simulink model "model_Asy_Motor_Control_PWM_v1"  (R2017b)
settings: Solver=ode45  StartTime=0.0  StopTime=3  MaxStep=1e-4  RelTol=1e-3
libraries: powerlib x8, dspstat3 x2, powerlib_meascontrol x1, simulink x1
settings Model: SimulationMode=accelerator  Creator=proso  LastModifiedBy=proso

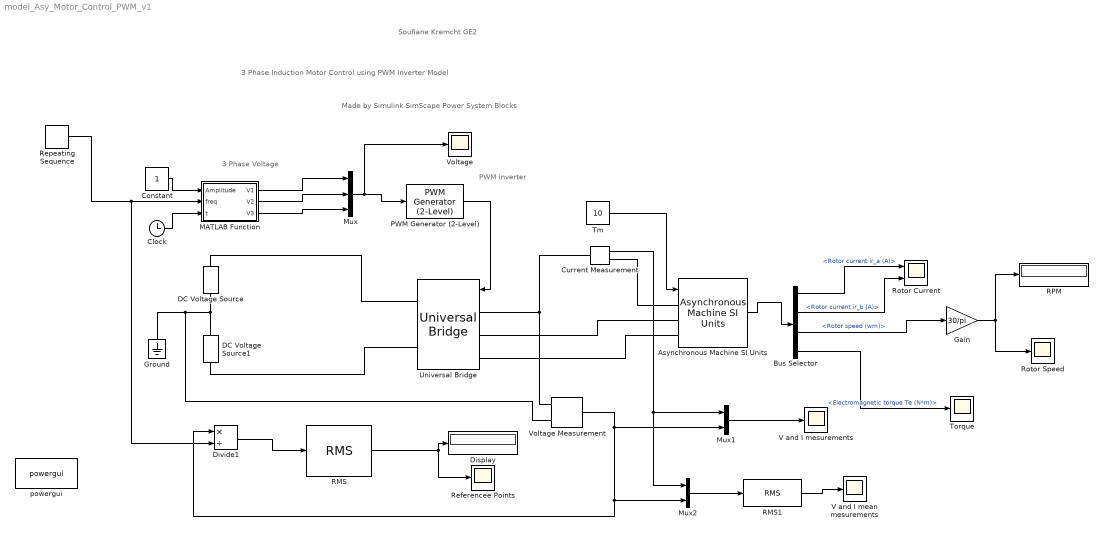
== system model_Asy_Motor_Control_PWM_v1 ==
  note: 3 Phase Voltage
  note: PWM inverter
  note: Soufiane Kremcht GE2
  note: Made by Simulink SimScape Power System Blocks
  note: 3 Phase Induction Motor Control using PWM Inverter Model
  Asynchronous Machine SI Units : powerlib/Machines/Asynchronous Machine SI Units  RotorType=Squirrel-cage  PresetModel="15:  5.4 HP (4KW)   400 V  50Hz 1430 RPM"  MechanicalLoad=Torque Tm  ShowDetailedParameters=on  ReferenceFrame=Rotor  Units=SI  MeasurementBus=off  NominalParameters=[4000 400 50]  Stator=[1.405 0.005839]  Rotor=[1.395 0.005839]  Cage1=[1.543 0.006067]  Cage2=[3.309 0.005654]  Lm=0.1722  Mechanical=[0.0131 0.002985 2]  PolePairs=2  InitialConditions=[0 0 0 0 0 0 0 0]  SimulateSaturation=off  Saturation=[14.03593122, 27.81365428, 53.79336849, 72.68890987, 97.98006896, 148.6815601, 215.7428561, 302.9841135, 428.7778367 ; 230, 322, 414, 460, 506, 552, 598, 644, 690]  LoadFlowParameters=1492000  TsPowergui=0  TsBlock=-1  IterativeModel=Trapezoidal non iterative  IterativeDiscreteModel=Trapezoidal non iterative  Pmec=1.492e+006
  Bus Selector : BusSelector  OutputSignals=Rotor measurements.Rotor current ir_a (A),Rotor measurements.Rotor current ir_b (A),Mechanical.Rotor speed (wm),Mechanical.Electromagnetic torque Te (N*m)
  Clock : Clock
  Constant : Constant
  Current Measurement : powerlib/Measurements/Current Measurement  PhasorSimulation=off  OutputType=Complex  PSBequivalent=0
  DC Voltage Source : powerlib/Electrical Sources/DC Voltage Source  Amplitude=100  Measurements=None
  DC Voltage Source1 : powerlib/Electrical Sources/DC Voltage Source  Amplitude=100  Measurements=None
  Display : Display
  Divide1 : Product  Inputs=*/
  Gain : Gain  Gain=30/pi
  Ground : powerlib/Elements/Ground  LConnTagsString=a
  MATLAB Function : MATLAB Function  TreatAsAtomicUnit=on
  Mux : Mux  Inputs=3
  Mux1 : Mux  Inputs=2
  Mux2 : Mux  Inputs=2
  PWM Generator (2-Level) : powerlib_meascontrol/Pulse & Signal Generators/PWM Generator (2-Level)  ModulatorType=Three-phase bridge (6 pulses)  ModulatorMode=Unsynchronized  Fc=27*60  Pc=90  nF=27  MinMax="[ -1  1 ]"  SamplingTechnique=Natural  ModulatingSignals=off  m=0.8  Freq=60  Phase=0  Ts=0  ShowCarrierOutport=off
      settings: SourceProductName=Simscape Power Systems
  RMS : dspstat3/RMS  run=off  directionMode=Each column  dimension=1  InputProcessing=Columns as channels (frame based)  reset_popup=None
  RMS1 : dspstat3/RMS  run=off  directionMode=Each column  dimension=1  InputProcessing=Columns as channels (frame based)  reset_popup=None
  RPM : Display
  Referencee Points : Scope
  Repeating Sequence : simulink/Sources/Repeating Sequence  rep_seq_t="[0 1 1.0001 2  2.0003 3]"  rep_seq_y=[10 10 20 20 20 30]
  Rotor Current : Scope  NumInputPorts=2
  Rotor Speed : Scope
  Tm : Constant  Value=10
  "Torque " : Scope
  Universal Bridge : powerlib/Power Electronics/Universal Bridge  Arms=3  SnubberResistance=1e5  SnubberCapacitance=inf  Device=IGBT / Diodes  Ron=1e-3  Lon=0  ForwardVoltages="[  0  0  ]"  ForwardVoltage=0  GTOparameters=[ 10e-6 , 20e-6 ]  IGBTparameters=[ 1e-6 , 2e-6 ]  Measurements=None  Measurements_2=None  converterType=Rectifier
  V and I mean mesurements : Scope
  V and I mesurements : Scope
  Voltage : Scope
  Voltage Measurement : powerlib/Measurements/Voltage Measurement  PhasorSimulation=off  OutputType=Complex  PSBequivalent=0
  powergui : powerlib/powergui  Priority=1  SimulationMode=Discrete  SampleTime=10e-5  frequency=60  Iterations=50  frequencyindice=50  Pbase=100e6  ErrMax=1e-4  UnitsV=kV  UnitsW=MW  buscounter=0  FunctionMessages=off  echomessages=off  EnableUseOfTLC=off  CurrentSourceSwitches=off  DisableSnubberDevices=off  DisableRonSwitches=off  DisableVfSwitches=off  DisplayEquations=off  SolverType=Tustin/Backward Euler (TBE)  Interpol=off  ExternalGateDelay=off  methode=off  Ts=100  x0status=blocks  SPID=on  SwTol=0  HookPort=off  RestoreLinks=warning  ResistiveCurrentMeasurement=off  Frange=[0:2:500]  Ylog=off  Xlog=on  ShowGrid=off  save=off  variable=ZData  structure=0  ZoomFFT=off  StartTime=0.0  cycles=1  DisplayStyle=1  fundamental=60  FreqAxis=off  MaxFrequency=1000  frequencyindicesteady=1  RmsSteady=1  display=off
  wires:
  Asynchronous Machine SI Units/1 -> Bus Selector/1
  Mux/1 -> Voltage/1, PWM Generator (2-Level)/1
  PWM Generator (2-Level)/1 -> Universal Bridge/1
  RMS/1 -> Display/1, Referencee Points/1
  Bus Selector/1 -> Rotor Current/1  "<Rotor current ir_a (A)>"
  Bus Selector/2 -> Rotor Current/2  "<Rotor current ir_b (A)>"
  Bus Selector/4 -> "Torque "/1  "<Electromagnetic torque Te (N*m)>"
  Voltage Measurement/1 -> Divide1/1, Mux2/2, Mux1/2
  Current Measurement/1 -> Mux2/1, Mux1/1
  Tm/1 -> Asynchronous Machine SI Units/1
  Mux1/1 -> V and I mesurements/1
  Divide1/1 -> RMS/1
  Mux2/1 -> RMS1/1
  RMS1/1 -> V and I mean mesurements/1
  Constant/1 -> MATLAB Function/1(Amplitude)
  Clock/1 -> MATLAB Function/3(t)
  MATLAB Function/1(V1) -> Mux/1
  MATLAB Function/2(V2) -> Mux/2
  MATLAB Function/3(V3) -> Mux/3
  Repeating Sequence/1 -> Divide1/2, MATLAB Function/2(freq)
  Gain/1 -> RPM/1, Rotor Speed/1
  Bus Selector/3 -> Gain/1  "<Rotor speed (wm)>"
  connections:
  Universal Bridge/LConn1 -- Current Measurement/LConn1 -- Voltage Measurement/LConn1
  Universal Bridge/LConn2 -- Asynchronous Machine SI Units/LConn2
  Universal Bridge/LConn3 -- Asynchronous Machine SI Units/LConn3
  Universal Bridge/RConn1 -- DC Voltage Source/RConn1
  DC Voltage Source/LConn1 -- Voltage Measurement/LConn2 -- Ground/LConn1 -- DC Voltage Source1/RConn1
  DC Voltage Source1/LConn1 -- Universal Bridge/RConn2
  Current Measurement/RConn1 -- Asynchronous Machine SI Units/LConn1

== matlab function model_Asy_Motor_Control_PWM_v1/MATLAB Function ==
  data: Amplitude input; V1 output; V2 output; V3 output; freq input; t input
function [V1,V2,V3]  = fcn(Amplitude,freq,t)
V1=Amplitude*sin(freq*2*pi*t);
V2=Amplitude*sin(freq*2*pi*t - 2*pi/3);
V3=Amplitude*sin(freq*pi*t + 2*pi/3);
